simulink model "hex_simplify_hex"  (R2017a)
settings: Solver=VariableStepAuto  StartTime=0.0  StopTime=10.0  RelTol=1e-3
undefined symbols (not defined in the file): sigbuilder_block, smiData, X, Y, Z
libraries: sm_lib x20, nesl_utility x19, simulink x1
(part 2 of 2)

== matlab function hex_simplify_hex/N(theta,dtheta)1/MATLAB Function1 ==
  data: q1 input; N1 output; q2 input; N2 output; N3 output; q3 input; qd1 input; qd2 input; qd3 input
function [N1, N2, N3] = fcn(q1,q2,q3,qd1,qd2,qd3)


l1 = 0.0285; l2 = 0.0758; l3 = 0.1298;
%q1 = 2; q2 = 0; q3 = pi/8;
%qd1 = 0.1; qd2 = 0.1; qd3 = 0.1;
%qdd1 = 0.1; qdd1 = 9; qdd1 = 0.01;
lc1 = l1/2; lc2 = l2/2; lc3 = l3/2;

Ixx1 = 0.000; Ixx2 = 0.000; Ixx3 = 0.000;
Iyy1 = 0.000; Iyy2 = 0.000; Iyy3 = 0.000;
Izz1 = 0.000; Izz2 = 0.000; Izz3 = 0.0000;

gx = 0;
gy = 0;
gz = 9.81;
m1 = 2; m2 = 2; m3 = 2;

Fx = 0;
Fy = 0;
Fz = 0;
b1 = 0.1; b2 = 0.1; b3 = 0.1; 

N1 = - Fz*l1  + b1*qd1 - Fz*l3*cos(q2 + q3) - Fz*l2*cos(q2) + (gy*lc3*m3*cos(q2 - q1 + q3))/2 + (gx*lc3*m3*sin(q2 - q1 + q3))/2 + (gy*l2*m3*cos(q1 + q2))/2 + (gy*lc2*m2*cos(q1 + q2))/2 - (gx*l2*m3*sin(q1 + q2))/2 - (gx*lc2*m2*sin(q1 + q2))/2 + gy*l1*m2*cos(q1) + gy*l1*m3*cos(q1) + gy*lc1*m1*cos(q1) - gx*l1*m2*sin(q1) - gx*l1*m3*sin(q1) - gx*lc1*m1*sin(q1) + (gy*l2*m3*cos(q1 - q2))/2 + (gy*lc2*m2*cos(q1 - q2))/2 - (gx*l2*m3*sin(q1 - q2))/2 - (gx*lc2*m2*sin(q1 - q2))/2 + (gy*lc3*m3*cos(q1 + q2 + q3))/2 - (gx*lc3*m3*sin(q1 + q2 + q3))/2 + Ixx2*qd1*qd2*sin(2*q2) - Iyy2*qd1*qd2*sin(2*q2) + Ixx3*qd1*qd2*sin(2*q2 + 2*q3) + Ixx3*qd1*qd3*sin(2*q2 + 2*q3) - Iyy3*qd1*qd2*sin(2*q2 + 2*q3) - Iyy3*qd1*qd3*sin(2*q2 + 2*q3)  - l2^2*m3*qd1*qd2*sin(2*q2) - lc2^2*m2*qd1*qd2*sin(2*q2)   - lc3^2*m3*qd1*qd2*sin(2*q2 + 2*q3) - lc3^2*m3*qd1*qd3*sin(2*q2 + 2*q3) - 2*l1*lc3*m3*qd1*qd2*sin(q2 + q3) - 2*l1*lc3*m3*qd1*qd3*sin(q2 + q3) - 2*l1*l2*m3*qd1*qd2*sin(q2) - 2*l1*lc2*m2*qd1*qd2*sin(q2) - l2*lc3*m3*qd1*qd3*sin(q3) - 2*l2*lc3*m3*qd1*qd2*sin(2*q2 + q3) - l2*lc3*m3*qd1*qd3*sin(2*q2 + q3);
N2 = Fy*l3 + b2*qd2 - (Ixx2*qd1^2*sin(2*q2))/2 + (Iyy2*qd1^2*sin(2*q2))/2 + Fy*l2*cos(q3) - (Ixx3*qd1^2*sin(2*q2 + 2*q3))/2 + (Iyy3*qd1^2*sin(2*q2 + 2*q3))/2 + Fx*l2*sin(q3) - (gy*lc3*m3*cos(q2 - q1 + q3))/2 - (gx*lc3*m3*sin(q2 - q1 + q3))/2 + (gy*l2*m3*cos(q1 + q2))/2 + (gy*lc2*m2*cos(q1 + q2))/2 + gz*lc3*m3*cos(q2 + q3) - (gx*l2*m3*sin(q1 + q2))/2 - (gx*lc2*m2*sin(q1 + q2))/2 + gz*l2*m3*cos(q2) + gz*lc2*m2*cos(q2) - (gy*l2*m3*cos(q1 - q2))/2 - (gy*lc2*m2*cos(q1 - q2))/2 + (l2^2*m3*qd1^2*sin(2*q2))/2 + (lc2^2*m2*qd1^2*sin(2*q2))/2 + (gx*l2*m3*sin(q1 - q2))/2 + (gx*lc2*m2*sin(q1 - q2))/2 + (gy*lc3*m3*cos(q1 + q2 + q3))/2 - (gx*lc3*m3*sin(q1 + q2 + q3))/2 + (lc3^2*m3*qd1^2*sin(2*q2 + 2*q3))/2 + l1*lc3*m3*qd1^2*sin(q2 + q3) + l1*l2*m3*qd1^2*sin(q2) + l1*lc2*m2*qd1^2*sin(q2) - l2*lc3*m3*qd3^2*sin(q3) + l2*lc3*m3*qd1^2*sin(2*q2 + q3) - 2*l2*lc3*m3*qd2*qd3*sin(q3);
N3 = Fy*l3 + b3*qd3 - (Ixx3*qd1^2*sin(2*q2 + 2*q3))/2 + (Iyy3*qd1^2*sin(2*q2 + 2*q3))/2 - (gy*lc3*m3*cos(q2 - q1 + q3))/2 - (gx*lc3*m3*sin(q2 - q1 + q3))/2 + gz*lc3*m3*cos(q2 + q3) + (gy*lc3*m3*cos(q1 + q2 + q3))/2 - (gx*lc3*m3*sin(q1 + q2 + q3))/2 + (lc3^2*m3*qd1^2*sin(2*q2 + 2*q3))/2 + l1*lc3*m3*qd1^2*sin(q2 + q3) + (l2*lc3*m3*qd1^2*sin(q3))/2 + l2*lc3*m3*qd2^2*sin(q3) + (l2*lc3*m3*qd1^2*sin(2*q2 + q3))/2 ;
